simulink subsystem "simscape_thermofluids_full_subsystem"  (R2024b)
settings: Solver=VariableStepAuto  StartTime=0.0  StopTime=10.0  RelTol=1e-3
values from neighbouring files (symbols this model uses):
  Ambient_temp = 300    [design_details.m]
  hose_length = 20    [design_details.m]
  Initial_temp = 300    [design_details.m]
  mass_per_length_supply = steel_density*wall_thickness*(supply_pipe_inner_area + supply_pipe_outer_area)    [design_details.m]
  return_pipe_inner_diameter = 0.1    [design_details.m]
  supply_pipe_inner_diameter = 0.05    [design_details.m]
  wall_thickness = 2/1000    (= 0.002)    [design_details.m]
undefined symbols (not defined in the file or in its folder): AC_Bypass_SOV_POS, AC_Engine_SOV_POS, AC_Return_SOV_POS, AC_Supply_SOV_POS, GH2_PROP_VALVE_POS, GS_GH2_SOV_POS, GS_RETURN_PROP_POS, GS_Return_SOV_POS, GS_Supply_SOV_POS, LH2_PROP_VALVE_POS, P_BYPASS, P_COUPLING_AC, P_COUPLING_AC_RETURN, P_COUPLINGS_GS, P_ENGINE_FEED, P_GH2_SUPPLY_GS, P_HOSE_GS, P_HOSE_RETURN_GS, P_PUMP_GS, P_SOV_RETURN_GS, P_TANK_AC, P_TANK_GS, P_VALVE_GS, T_BYPASS, T_COUPLING_AC, T_COUPLING_AC_RETURN, T_COUPLINGS_GS, T_ENGINE_FEED, T_GH2_SUPPLY_GS, T_HOSE_GS, T_HOSE_RETURN_GS, T_PUMP_GS, T_SOV_RETURN_GS, T_TANK_AC, T_TANK_GS, T_VALVE_GS
libraries: fl_lib x55, nesl_utility x54, SimscapeFluids_lib x10
(part 2 of 2)

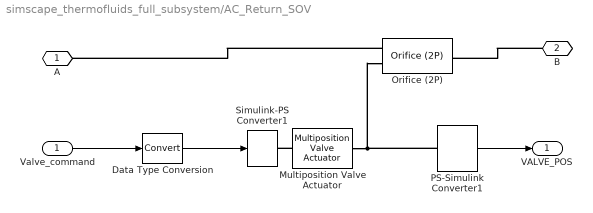
== system simscape_thermofluids_full_subsystem/AC_Return_SOV ==
  Valve_command : Inport
  Data Type Conversion : DataTypeConversion  SaturateOnIntegerOverflow=off  RndMeth=Floor
  Multiposition Valve Actuator : SimscapeFluids_lib/Valve Actuators/Multiposition Valve Actuator  positions=fluids.valve_actuators.enum.actuator_num_positions.two  stroke=3e-2 m  t_on=1 s  t_off=1 s  act_signal=0.5  init_position_2=fluids.valve_actuators.enum.actuator_two_pos_ic.retracted  init_position_3=fluids.valve_actuators.enum.actuator_three_pos_ic.neutral  act_orientation=simscape.enum.posneg.positive  local_time_specify=off  local_time_priority=None  local_time=0 s  local_time_nominal_specify=off  local_time_nominal_value=1  local_time_nominal_unit=s
      settings: InternalSimscapePortConfiguration="{\"Bottom\":[],\"Left\":[{\"id\":\"A\",\"label\":\"A\",\"type\":\"input\"}],\"Right\":[{\"id\":\"S\",\"label\":\"S\",\"type\":\"output\"}],\"Top\":[]}"
  Orifice (2P) : SimscapeFluids_lib/Two-Phase Fluid/Valves & Orifices/Orifice (2P)  orifice_type=foundation.enum.constant_variable.variable  constant_liquid_orifice_parameterization=fluids.two_phase_fluid.valves_orifices.enum.LiquidConstantOrificeParameterization.Area  variable_liquid_orifice_parameterization=fluids.two_phase_fluid.valves_orifices.enum.LiquidOrificeParameterization.LinearArea  mdot_nominal_constant=0.1 kg/s  delta_p_nominal_constant=0.001 MPa  orifice_area_constant=1e-4 m^2  S_min=0 m  del_S=3e-2 m  open_orientation=fluids.two_phase_fluid.valves_orifices.enum.OrificeOrientation.Positive  mdot_nominal_max=0.1 kg/s  delta_p_nominal_max=0.001 MPa  orifice_area_max=AC_return_valve_orifice_area m^2  S_TLU=[0, .002, .004, .007, .017] m  orifice_area_TLU=[1e-10, 2e-05, 4e-05, 6e-05, 8e-05, .0001] m^2  energy_spec=foundation.enum.energy_spec.temperature  p_inlet=0.101325 MPa  T_inlet=293.15 K  x_inlet=0  alpha_inlet=0  h_inlet=400 kJ/kg  u_inlet=400 kJ/kg  Cd=AC_return_valve_discharge_coeff  pressure_recovery=false  leakage_fraction=1e-6  smoothing_factor=0.01  B_lam=0.999  tau_x=0.1 s  area=AC_return_line_port_inner_area m^2  vapor_orifice_parameterization=fluids.two_phase_fluid.valves_orifices.enum.VaporOrificeParameterization.Cv  opening_characteristic=fluids.two_phase_fluid.valves_orifices.enum.OpeningCharacteristics.Linear  Cv_constant=4  Cv_max=4  S_Cv_TLU=[0, .003, .006, .009, .012, .015] m  Cv_TLU=[1e-06, .8, 1.6, 2.4, 3.2, 4]  xT_Cv=0.7  Kv_constant=3.6  Kv_max=3.6  S_Kv_TLU=[0, .003, .006, .009, .012, .015] m  Kv_TLU=[1e-06, .72, 1.44, 2.16, 2.88, 3.6]  xT_Kv=0.7  S_orifice_area_TLU=[0, .003, .006, .009, .012, .015] m
      settings: InternalSimscapePortConfiguration="{\"Bottom\":[],\"Left\":[{\"id\":\"A\",\"label\":\"A\",\"type\":\"foundation.two_phase_fluid.two_phase_fluid\"},{\"id\":\"S\",\"label\":\"S\",\"type\":\"input\"}],\"Right\":[{\"id\":\"B\",\"label\":\"B\",\"type\":\"foundation.two_phase_fluid.two_phase_fluid\"}],\"Top\":[]}"
  PS-Simulink Converter1 : nesl_utility/PS-Simulink Converter  PhysicalDomain=network_engine_domain  SubClassName=ps_output  LeftPortType=input  RightPortType=output  PseudoPeriodic=off  Frequencies=[]  VectorFormat=inherit  Unit=inherit  AffineConversion=off
  Simulink-PS Converter1 : nesl_utility/Simulink-PS Converter  PhysicalDomain=network_engine_domain  SubClassName=ps_input  LeftPortType=input  RightPortType=output  PseudoPeriodic=off  Frequencies=[]  NoiseDistribution=none  NoiseParameters=[]  Unit=1  AffineConversion=off  FilteringAndDerivatives=zero  SimscapeFilterOrder=1  InputFilterTimeConstant=0.001  UdotUserProvided=1
  A : PMIOPort  Side=Left
  B : PMIOPort  Port=2  Side=Right
  VALVE_POS : Outport
  wires:
  PS-Simulink Converter1/1 -> VALVE_POS/1
  Data Type Conversion/1 -> Simulink-PS Converter1/1
  Valve_command/1 -> Data Type Conversion/1
  connections:
  B/RConn1 -- Orifice (2P)/RConn1
  Orifice (2P)/LConn1 -- A/RConn1
  Multiposition Valve Actuator/LConn1 -- Simulink-PS Converter1/RConn1
  PS-Simulink Converter1/LConn1 -- Orifice (2P)/LConn2 -- Multiposition Valve Actuator/RConn1

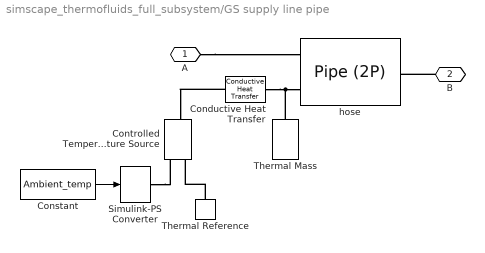
== system simscape_thermofluids_full_subsystem/GS supply line pipe ==
  Conductive Heat Transfer : fl_lib/Thermal/Thermal Elements/Conductive Heat Transfer  thermal_type=foundation.enum.ConstantVariableTabulated.Constant  wall_geometry=foundation.enum.ConductionWallGeometry.Cylindrical  area=hose_length m^2  thickness=0.01 m  d_in=supply_pipe_inner_diameter m  d_out=wall_thickness*2 + supply_pipe_inner_diameter m  L=2 m  th_cond_min=10 W/(K*m)  th_cond=pipe_thermal_conductivity W/(m*K)  th_cond_TLU=[413, 401, 392, 383, 371, 357, 342] W/(K*m)  temp_TLU=[200, 273, 400, 600, 800, 1000, 1200] K  T_specify=off  T_priority=None  T=0 K  T_nominal_specify=off  T_nominal_value=1  T_nominal_unit=K  Q_specify=off  Q_priority=None  Q=0 W  Q_nominal_specify=off  Q_nominal_value=1  Q_nominal_unit=W
  Constant : Constant  Value=Ambient_temp
  Controlled Temperature Source : fl_lib/Thermal/Thermal Sources/Controlled Temperature Source
  Simulink-PS Converter : nesl_utility/Simulink-PS Converter  PhysicalDomain=network_engine_domain  SubClassName=ps_input  LeftPortType=input  RightPortType=output  PseudoPeriodic=off  Frequencies=[]  NoiseDistribution=none  NoiseParameters=[]  Unit=1  AffineConversion=off  FilteringAndDerivatives=zero  SimscapeFilterOrder=1  InputFilterTimeConstant=0.001  UdotUserProvided=1
  Thermal Mass : fl_lib/Thermal/Thermal Elements/Thermal Mass  mass_type=foundation.enum.constant_variable.constant  mass=mass_per_length_supply*2 kg  sp_heat=250 J/kg/K  mass_min=1e-6 kg  num_ports=foundation.enum.numPorts2.one  m_specify=off  m_priority=High  m=1 kg  m_nominal_specify=off  m_nominal_value=1  m_nominal_unit=kg  T_specify=on  T_priority=High  T=20 K  T_nominal_specify=off  T_nominal_value=1  T_nominal_unit=K  Q_specify=off  Q_priority=None  Q=0 W  Q_nominal_specify=off  Q_nominal_value=1  Q_nominal_unit=W
  Thermal Reference : fl_lib/Thermal/Thermal Elements/Thermal Reference
  hose : fl_lib/Two-Phase Fluid/Elements/Pipe (2P)  length=2 m  area=supply_pipe_inner_area m^2  Dh=supply_pipe_inner_diameter m  length_add=0.1 m  roughness=15e-6 m  Re_lam=2000  Re_tur=4000  shape_factor=64  Nu_lam=3.66  inertia=false  energy_spec=foundation.enum.energy_spec.temperature  p_init=1.5 bar  T_init=20 K  x_init=0.5  alpha_init=0.5  h_init=1500 kJ/kg  u_init=1500 kJ/kg  mdot_init=0 kg/s  time_constant=0.1 s
      settings: InternalSimscapePortConfiguration="{\"Bottom\":[],\"Left\":[{\"id\":\"A\",\"label\":\"A\",\"type\":\"foundation.two_phase_fluid.two_phase_fluid\"},{\"id\":\"H\",\"label\":\"H\",\"type\":\"foundation.thermal.thermal\"}],\"Right\":[{\"id\":\"B\",\"label\":\"B\",\"type\":\"foundation.two_phase_fluid.two_phase_fluid\"}],\"Top\":[]}"
  A : PMIOPort  Side=Left
  B : PMIOPort  Port=2  Side=Right
  wires:
  Constant/1 -> Simulink-PS Converter/1
  connections:
  B/RConn1 -- hose/RConn1
  A/RConn1 -- hose/LConn1
  Thermal Reference/LConn1 -- Controlled Temperature Source/RConn2
  Simulink-PS Converter/RConn1 -- Controlled Temperature Source/RConn1
  Conductive Heat Transfer/LConn1 -- Controlled Temperature Source/LConn1
  Conductive Heat Transfer/RConn1 -- hose/LConn2 -- Thermal Mass/LConn1

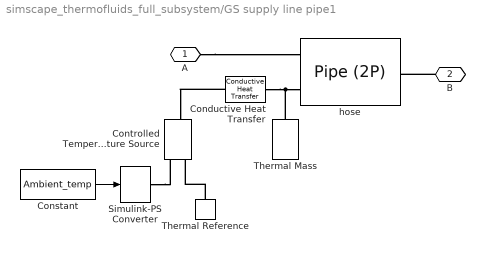
== system simscape_thermofluids_full_subsystem/GS supply line pipe1 ==
  Conductive Heat Transfer : fl_lib/Thermal/Thermal Elements/Conductive Heat Transfer  thermal_type=foundation.enum.ConstantVariableTabulated.Constant  wall_geometry=foundation.enum.ConductionWallGeometry.Cylindrical  area=hose_length m^2  thickness=0.01 m  d_in=supply_pipe_inner_diameter m  d_out=wall_thickness*2 + supply_pipe_inner_diameter m  L=2 m  th_cond_min=10 W/(K*m)  th_cond=pipe_thermal_conductivity W/(m*K)  th_cond_TLU=[413, 401, 392, 383, 371, 357, 342] W/(K*m)  temp_TLU=[200, 273, 400, 600, 800, 1000, 1200] K  T_specify=off  T_priority=None  T=0 K  T_nominal_specify=off  T_nominal_value=1  T_nominal_unit=K  Q_specify=off  Q_priority=None  Q=0 W  Q_nominal_specify=off  Q_nominal_value=1  Q_nominal_unit=W
  Constant : Constant  Value=Ambient_temp
  Controlled Temperature Source : fl_lib/Thermal/Thermal Sources/Controlled Temperature Source
  Simulink-PS Converter : nesl_utility/Simulink-PS Converter  PhysicalDomain=network_engine_domain  SubClassName=ps_input  LeftPortType=input  RightPortType=output  PseudoPeriodic=off  Frequencies=[]  NoiseDistribution=none  NoiseParameters=[]  Unit=1  AffineConversion=off  FilteringAndDerivatives=zero  SimscapeFilterOrder=1  InputFilterTimeConstant=0.001  UdotUserProvided=1
  Thermal Mass : fl_lib/Thermal/Thermal Elements/Thermal Mass  mass_type=foundation.enum.constant_variable.constant  mass=mass_per_length_supply*2 kg  sp_heat=250 J/kg/K  mass_min=1e-6 kg  num_ports=foundation.enum.numPorts2.one  m_specify=off  m_priority=High  m=1 kg  m_nominal_specify=off  m_nominal_value=1  m_nominal_unit=kg  T_specify=on  T_priority=High  T=Ambient_temp K  T_nominal_specify=off  T_nominal_value=1  T_nominal_unit=K  Q_specify=off  Q_priority=None  Q=0 W  Q_nominal_specify=off  Q_nominal_value=1  Q_nominal_unit=W
  Thermal Reference : fl_lib/Thermal/Thermal Elements/Thermal Reference
  hose : fl_lib/Two-Phase Fluid/Elements/Pipe (2P)  length=2 m  area=supply_pipe_inner_area m^2  Dh=supply_pipe_inner_diameter m  length_add=0.1 m  roughness=15e-6 m  Re_lam=2000  Re_tur=4000  shape_factor=64  Nu_lam=3.66  inertia=false  energy_spec=foundation.enum.energy_spec.temperature  p_init=1.5 bar  T_init=Ambient_temp K  x_init=0.5  alpha_init=0.5  h_init=1500 kJ/kg  u_init=1500 kJ/kg  mdot_init=0 kg/s  time_constant=0.1 s
      settings: InternalSimscapePortConfiguration="{\"Bottom\":[],\"Left\":[{\"id\":\"A\",\"label\":\"A\",\"type\":\"foundation.two_phase_fluid.two_phase_fluid\"},{\"id\":\"H\",\"label\":\"H\",\"type\":\"foundation.thermal.thermal\"}],\"Right\":[{\"id\":\"B\",\"label\":\"B\",\"type\":\"foundation.two_phase_fluid.two_phase_fluid\"}],\"Top\":[]}"
  A : PMIOPort  Side=Left
  B : PMIOPort  Port=2  Side=Right
  wires:
  Constant/1 -> Simulink-PS Converter/1
  connections:
  B/RConn1 -- hose/RConn1
  A/RConn1 -- hose/LConn1
  Thermal Reference/LConn1 -- Controlled Temperature Source/RConn2
  Simulink-PS Converter/RConn1 -- Controlled Temperature Source/RConn1
  Conductive Heat Transfer/LConn1 -- Controlled Temperature Source/LConn1
  Conductive Heat Transfer/RConn1 -- hose/LConn2 -- Thermal Mass/LConn1

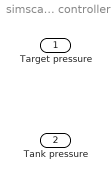
== system simscape_thermofluids_full_subsystem/GS tank pressure controller ==
  Target pressure : Inport
  Tank pressure : Inport  Port=2

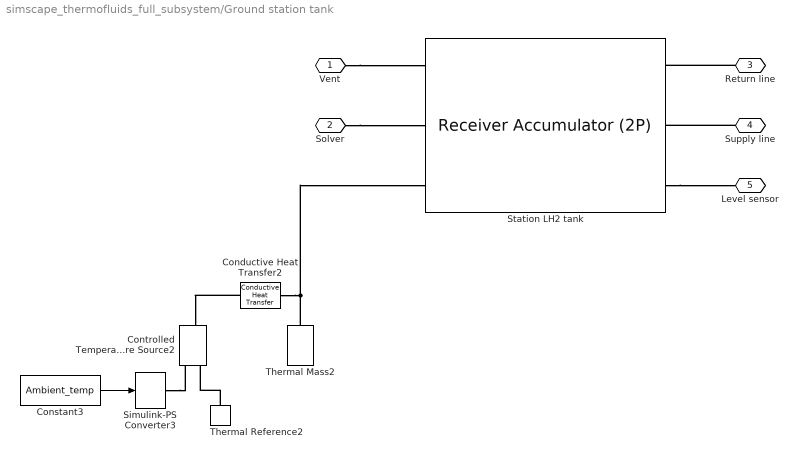
== system simscape_thermofluids_full_subsystem/Ground station tank ==
  Conductive Heat Transfer2 : fl_lib/Thermal/Thermal Elements/Conductive Heat Transfer  thermal_type=foundation.enum.ConstantVariableTabulated.Constant  wall_geometry=foundation.enum.ConductionWallGeometry.Planar  area=10 m^2  thickness=0.01 m  d_in=0.05 m  d_out=0.1 m  L=1 m  th_cond_min=10 W/(K*m)  th_cond=0.001 W/(m*K)  th_cond_TLU=[413, 401, 392, 383, 371, 357, 342] W/(K*m)  temp_TLU=[200, 273, 400, 600, 800, 1000, 1200] K  T_specify=off  T_priority=None  T=0 K  T_nominal_specify=off  T_nominal_value=1  T_nominal_unit=K  Q_specify=off  Q_priority=None  Q=0 W  Q_nominal_specify=off  Q_nominal_value=1  Q_nominal_unit=W
  Constant3 : Constant  Value=Ambient_temp
  Controlled Temperature Source2 : fl_lib/Thermal/Thermal Sources/Controlled Temperature Source
  Simulink-PS Converter3 : nesl_utility/Simulink-PS Converter  PhysicalDomain=network_engine_domain  SubClassName=ps_input  LeftPortType=input  RightPortType=output  PseudoPeriodic=off  Frequencies=[]  NoiseDistribution=none  NoiseParameters=[]  Unit=1  AffineConversion=off  FilteringAndDerivatives=zero  SimscapeFilterOrder=1  InputFilterTimeConstant=0.001  UdotUserProvided=1
  Station LH2 tank : SimscapeFluids_lib/Two-Phase Fluid/Tanks & Accumulators/Receiver Accumulator (2P)  volume=10 m^3  tank_area=2 m^2  area_AV=0.02 m^2  area_BV=return_pipe_inner_area m^2  area_AL=supply_pipe_inner_area m^2  area_BL=supply_pipe_inner_area m^2  V_frac_liq_error=simscape.enum.assert.action.none  V_frac_liq_min=0.05  V_frac_liq_max=0.95  V_frac_smooth=0.05  p_crit_error=simscape.enum.assert.action.error  hc_vap=20 W/(K*m^2)  hc_liq=100 W/(K*m^2)  p_init=3 bar  fraction_spec=fluids.two_phase_fluid.tanks_accumulators.enum.LiquidFractionSpec.Volume  M_frac_liq_init=0.5  V_frac_liq_init=0.9  saturated_init=false  energy_spec=fluids.two_phase_fluid.tanks_accumulators.enum.EnergySpec.Temperature  delta_T_sub_init=5 deltaK  delta_T_sup_init=5 deltaK  T_liq_init=20 K  T_vap_init=27 K  h_liq_init=400 kJ/kg  h_vap_init=2700 kJ/kg  u_liq_init=400 kJ/kg  u_vap_init=2700 kJ/kg  tau_vap_cond=0.1 s
      settings: InternalSimscapePortConfiguration="{\"Bottom\":[],\"Left\":[{\"id\":\"AV\",\"label\":\"AV\",\"type\":\"foundation.two_phase_fluid.two_phase_fluid\"},{\"id\":\"AL\",\"label\":\"AL\",\"type\":\"foundation.two_phase_fluid.two_phase_fluid\"},{\"id\":\"H\",\"label\":\"H\",\"type\":\"foundation.thermal.thermal\"}],\"Right\":[{\"id\":\"BV\",\"label\":\"BV\",\"type\":\"foundation.two_phase_fluid.two_phase_fluid\"},{\"id\":\"BL\",\"label\":\"BL\",\"type\":\"foundation.two_phase_fluid.two_phase_fluid\"},{\"id\":\"L\",\"label\":\"L\",\"type\":\"output\"}],\"Top\":[]}"
  Thermal Mass2 : fl_lib/Thermal/Thermal Elements/Thermal Mass  mass_type=foundation.enum.constant_variable.constant  mass=500 kg  sp_heat=473 J/kg/K  mass_min=1e-6 kg  num_ports=foundation.enum.numPorts2.one  m_specify=off  m_priority=High  m=1 kg  m_nominal_specify=off  m_nominal_value=1  m_nominal_unit=kg  T_specify=on  T_priority=High  T=20 K  T_nominal_specify=off  T_nominal_value=1  T_nominal_unit=K  Q_specify=off  Q_priority=None  Q=0 W  Q_nominal_specify=off  Q_nominal_value=1  Q_nominal_unit=W
  Thermal Reference2 : fl_lib/Thermal/Thermal Elements/Thermal Reference
  Vent : PMIOPort  Side=Left
  Solver : PMIOPort  Port=2  Side=Left
  Return line : PMIOPort  Port=3  Side=Right
  Supply line : PMIOPort  Port=4  Side=Right
  Level sensor : PMIOPort  Port=5  Side=Right
  wires:
  Constant3/1 -> Simulink-PS Converter3/1
  connections:
  Thermal Mass2/LConn1 -- Station LH2 tank/LConn3 -- Conductive Heat Transfer2/RConn1
  Conductive Heat Transfer2/LConn1 -- Controlled Temperature Source2/LConn1
  Simulink-PS Converter3/RConn1 -- Controlled Temperature Source2/RConn1
  Thermal Reference2/LConn1 -- Controlled Temperature Source2/RConn2
  Solver/RConn1 -- Station LH2 tank/LConn2
  Vent/RConn1 -- Station LH2 tank/LConn1
  Return line/RConn1 -- Station LH2 tank/RConn1
  Supply line/RConn1 -- Station LH2 tank/RConn2
  Station LH2 tank/RConn3 -- Level sensor/RConn1

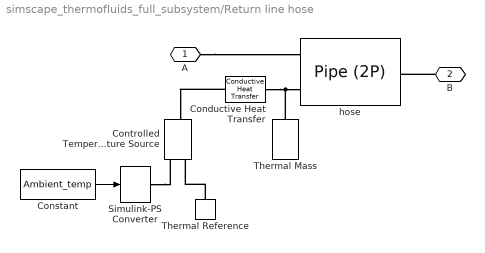
== system simscape_thermofluids_full_subsystem/Return line hose ==
  Conductive Heat Transfer : fl_lib/Thermal/Thermal Elements/Conductive Heat Transfer  thermal_type=foundation.enum.ConstantVariableTabulated.Constant  wall_geometry=foundation.enum.ConductionWallGeometry.Cylindrical  area=hose_length m^2  thickness=0.01 m  d_in=return_pipe_inner_diameter m  d_out=wall_thickness*2 + return_pipe_inner_diameter m  L=hose_length m  th_cond_min=10 W/(K*m)  th_cond=hose_thermal_conductivity W/(m*K)  th_cond_TLU=[413, 401, 392, 383, 371, 357, 342] W/(K*m)  temp_TLU=[200, 273, 400, 600, 800, 1000, 1200] K  T_specify=off  T_priority=None  T=0 K  T_nominal_specify=off  T_nominal_value=1  T_nominal_unit=K  Q_specify=off  Q_priority=None  Q=0 W  Q_nominal_specify=off  Q_nominal_value=1  Q_nominal_unit=W
  Constant : Constant  Value=Ambient_temp
  Controlled Temperature Source : fl_lib/Thermal/Thermal Sources/Controlled Temperature Source
  Simulink-PS Converter : nesl_utility/Simulink-PS Converter  PhysicalDomain=network_engine_domain  SubClassName=ps_input  LeftPortType=input  RightPortType=output  PseudoPeriodic=off  Frequencies=[]  NoiseDistribution=none  NoiseParameters=[]  Unit=1  AffineConversion=off  FilteringAndDerivatives=zero  SimscapeFilterOrder=1  InputFilterTimeConstant=0.001  UdotUserProvided=1
  Thermal Mass : fl_lib/Thermal/Thermal Elements/Thermal Mass  mass_type=foundation.enum.constant_variable.constant  mass=mass_per_length_supply*hose_length kg  sp_heat=467 J/kg/K  mass_min=1e-6 kg  num_ports=foundation.enum.numPorts2.one  m_specify=off  m_priority=High  m=1 kg  m_nominal_specify=off  m_nominal_value=1  m_nominal_unit=kg  T_specify=on  T_priority=High  T=Initial_temp K  T_nominal_specify=off  T_nominal_value=1  T_nominal_unit=K  Q_specify=off  Q_priority=None  Q=0 W  Q_nominal_specify=off  Q_nominal_value=1  Q_nominal_unit=W
  Thermal Reference : fl_lib/Thermal/Thermal Elements/Thermal Reference
  hose : fl_lib/Two-Phase Fluid/Elements/Pipe (2P)  length=hose_length m  area=supply_pipe_inner_area m^2  Dh=supply_pipe_inner_diameter m  length_add=0.1 m  roughness=15e-6 m  Re_lam=2000  Re_tur=4000  shape_factor=64  Nu_lam=3.66  inertia=false  energy_spec=foundation.enum.energy_spec.temperature  p_init=initial_hose_p bar  T_init=Initial_temp K  x_init=0.5  alpha_init=0.5  h_init=1500 kJ/kg  u_init=1500 kJ/kg  mdot_init=0 kg/s  time_constant=0.1 s
      settings: InternalSimscapePortConfiguration="{\"Bottom\":[],\"Left\":[{\"id\":\"A\",\"label\":\"A\",\"type\":\"foundation.two_phase_fluid.two_phase_fluid\"},{\"id\":\"H\",\"label\":\"H\",\"type\":\"foundation.thermal.thermal\"}],\"Right\":[{\"id\":\"B\",\"label\":\"B\",\"type\":\"foundation.two_phase_fluid.two_phase_fluid\"}],\"Top\":[]}"
  A : PMIOPort  Side=Left
  B : PMIOPort  Port=2  Side=Right
  wires:
  Constant/1 -> Simulink-PS Converter/1
  connections:
  hose/LConn2 -- Conductive Heat Transfer/RConn1 -- Thermal Mass/LConn1
  Conductive Heat Transfer/LConn1 -- Controlled Temperature Source/LConn1
  Simulink-PS Converter/RConn1 -- Controlled Temperature Source/RConn1
  Thermal Reference/LConn1 -- Controlled Temperature Source/RConn2
  A/RConn1 -- hose/LConn1
  B/RConn1 -- hose/RConn1

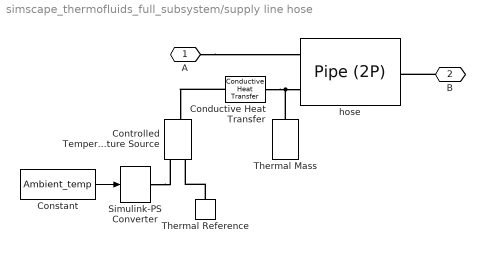
== system simscape_thermofluids_full_subsystem/supply line hose ==
  Conductive Heat Transfer : fl_lib/Thermal/Thermal Elements/Conductive Heat Transfer  thermal_type=foundation.enum.ConstantVariableTabulated.Constant  wall_geometry=foundation.enum.ConductionWallGeometry.Cylindrical  area=hose_length m^2  thickness=0.01 m  d_in=supply_pipe_inner_diameter m  d_out=wall_thickness*2 + supply_pipe_inner_diameter m  L=hose_length m  th_cond_min=10 W/(K*m)  th_cond=hose_thermal_conductivity W/(m*K)  th_cond_TLU=[413, 401, 392, 383, 371, 357, 342] W/(K*m)  temp_TLU=[200, 273, 400, 600, 800, 1000, 1200] K  T_specify=off  T_priority=None  T=0 K  T_nominal_specify=off  T_nominal_value=1  T_nominal_unit=K  Q_specify=off  Q_priority=None  Q=0 W  Q_nominal_specify=off  Q_nominal_value=1  Q_nominal_unit=W
  Constant : Constant  Value=Ambient_temp
  Controlled Temperature Source : fl_lib/Thermal/Thermal Sources/Controlled Temperature Source
  Simulink-PS Converter : nesl_utility/Simulink-PS Converter  PhysicalDomain=network_engine_domain  SubClassName=ps_input  LeftPortType=input  RightPortType=output  PseudoPeriodic=off  Frequencies=[]  NoiseDistribution=none  NoiseParameters=[]  Unit=1  AffineConversion=off  FilteringAndDerivatives=zero  SimscapeFilterOrder=1  InputFilterTimeConstant=0.001  UdotUserProvided=1
  Thermal Mass : fl_lib/Thermal/Thermal Elements/Thermal Mass  mass_type=foundation.enum.constant_variable.constant  mass=mass_per_length_supply*hose_length kg  sp_heat=250 J/kg/K  mass_min=1e-6 kg  num_ports=foundation.enum.numPorts2.one  m_specify=off  m_priority=High  m=1 kg  m_nominal_specify=off  m_nominal_value=1  m_nominal_unit=kg  T_specify=on  T_priority=High  T=Initial_temp K  T_nominal_specify=off  T_nominal_value=1  T_nominal_unit=K  Q_specify=off  Q_priority=None  Q=0 W  Q_nominal_specify=off  Q_nominal_value=1  Q_nominal_unit=W
  Thermal Reference : fl_lib/Thermal/Thermal Elements/Thermal Reference
  hose : fl_lib/Two-Phase Fluid/Elements/Pipe (2P)  length=hose_length m  area=supply_pipe_inner_area m^2  Dh=supply_pipe_inner_diameter m  length_add=0.1 m  roughness=15e-6 m  Re_lam=2000  Re_tur=4000  shape_factor=64  Nu_lam=3.66  inertia=false  energy_spec=foundation.enum.energy_spec.temperature  p_init=initial_hose_p bar  T_init=Initial_temp K  x_init=0.5  alpha_init=0.5  h_init=1500 kJ/kg  u_init=1500 kJ/kg  mdot_init=0 kg/s  time_constant=0.1 s
      settings: InternalSimscapePortConfiguration="{\"Bottom\":[],\"Left\":[{\"id\":\"A\",\"label\":\"A\",\"type\":\"foundation.two_phase_fluid.two_phase_fluid\"},{\"id\":\"H\",\"label\":\"H\",\"type\":\"foundation.thermal.thermal\"}],\"Right\":[{\"id\":\"B\",\"label\":\"B\",\"type\":\"foundation.two_phase_fluid.two_phase_fluid\"}],\"Top\":[]}"
  A : PMIOPort  Side=Left
  B : PMIOPort  Port=2  Side=Right
  wires:
  Constant/1 -> Simulink-PS Converter/1
  connections:
  hose/LConn2 -- Conductive Heat Transfer/RConn1 -- Thermal Mass/LConn1
  Conductive Heat Transfer/LConn1 -- Controlled Temperature Source/LConn1
  Simulink-PS Converter/RConn1 -- Controlled Temperature Source/RConn1
  Thermal Reference/LConn1 -- Controlled Temperature Source/RConn2
  A/RConn1 -- hose/LConn1
  B/RConn1 -- hose/RConn1
